simulink model "BVPmodel"  (R2016a)
settings: Solver=VariableStepAuto  StartTime=0.0  StopTime=10.0  RelTol=1e-3
settings Model: Creator=Bakry  LastModifiedBy=Bakry

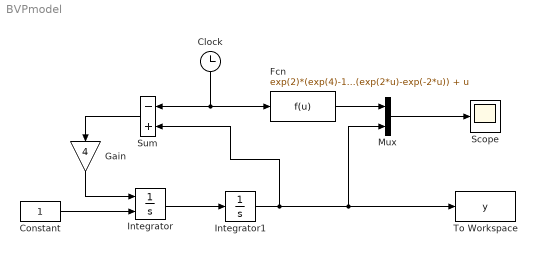
== system BVPmodel ==
  Clock : Clock
  Constant : Constant
  Fcn : Fcn  Expr=exp(2)*(exp(4)-1)*(exp(2*u)-exp(-2*u)) + u
  Gain : Gain  Gain=4
  Integrator : Integrator  InitialConditionSource=external
  Integrator1 : Integrator
  Mux : Mux  Inputs=2
  Scope : Scope
  Sum : Sum  Inputs=-+
  To Workspace : ToWorkspace  VariableName=y  SampleTime=-1
  wires:
  Clock/1 -> Fcn/1, Sum/1
  Fcn/1 -> Mux/1
  Mux/1 -> Scope/1
  Integrator/1 -> Integrator1/1
  Constant/1 -> Integrator/2
  Gain/1 -> Integrator/1
  Sum/1 -> Gain/1
  Integrator1/1 -> Sum/2, To Workspace/1, Mux/2
